simulink model "magnes_bb"  (R2015a)
settings: Solver=ode3  StartTime=0.0  StopTime=0.001  FixedStep=0.00001  RelTol=1e-3
settings Model: Creator=Student  LastModifiedBy=lenovo

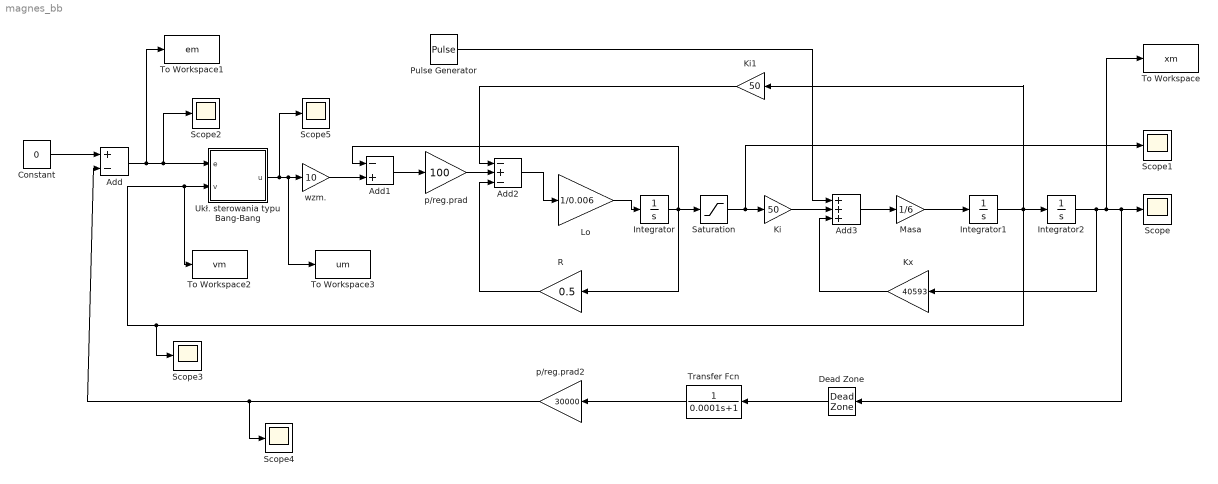
== system magnes_bb ==
  Add : Sum  Inputs=+-
  Add1 : Sum  Inputs=-+
  Add2 : Sum  Inputs=-+-
  Add3 : Sum  Inputs=+++
  Constant : Constant  Value=0
  Dead Zone : DeadZone  LowerValue=-1e-6  UpperValue=1e-6  SaturateOnIntegerOverflow=on
  Integrator : Integrator
  Integrator1 : Integrator
  Integrator2 : Integrator
  Ki : Gain  Gain=50
  Ki1 : Gain  Gain=50
  Kx : Gain  Gain=40593
  Lo : Gain  Gain=1/0.006
  Masa : Gain  Gain=1/6
  Pulse Generator : DiscretePulseGenerator  PulseType=Time based  Amplitude=6*9.81*0.5  Period=0.1  PulseWidth=50  PhaseDelay=0.2
  R : Gain  Gain=0.5
  Saturation : Saturate  UpperLimit=10  LowerLimit=-10
  Scope{,1..5} (6 alike) : Scope
      Scope settings: YMin=-1.5e-06  YMax=1.5e-06
      Scope2 settings: SaveName=ScopeData2
      Scope3 settings: SaveName=ScopeData3
      Scope4 settings: SaveName=ScopeData4
      Scope5 settings: YMin=0.85063  YMax=0.95303  SaveName=ScopeData5
  To Workspace : ToWorkspace  VariableName=xm  SaveFormat=Timeseries  SampleTime=-1
  To Workspace1 : ToWorkspace  VariableName=em  SaveFormat=Timeseries  SampleTime=-1
  To Workspace2 : ToWorkspace  VariableName=vm  SaveFormat=Timeseries  SampleTime=-1
  To Workspace3 : ToWorkspace  VariableName=um  SaveFormat=Timeseries  SampleTime=-1
  Transfer Fcn : TransferFcn  Denominator=[0.0001 1]
  Ukł. sterowania typu Bang-Bang : Stateflow chart  TreatAsAtomicUnit=on
  p/reg.prad : Gain  Gain=100
  p/reg.prad2 : Gain  Gain=30000
  wzm. : Gain  Gain=10
  wires:
  wzm./1 -> Add1/2
  Add1/1 -> p/reg.prad/1
  Add2/1 -> Lo/1
  p/reg.prad/1 -> Add2/2
  Lo/1 -> Integrator/1
  Integrator/1 -> R/1, Add1/1, Saturation/1
  R/1 -> Add2/3
  Constant/1 -> Add/1
  Add/1 -> To Workspace1/1, Scope2/1, Ukł. sterowania typu Bang-Bang/1(e)
  Saturation/1 -> Scope1/1, Ki/1
  Ki/1 -> Add3/2
  Add3/1 -> Masa/1
  Masa/1 -> Integrator1/1
  Kx/1 -> Add3/3
  Dead Zone/1 -> Transfer Fcn/1
  Transfer Fcn/1 -> p/reg.prad2/1
  p/reg.prad2/1 -> Scope4/1, Add/2
  Integrator2/1 -> Kx/1, To Workspace/1, Dead Zone/1, Scope/1
  Integrator1/1 -> Scope3/1, To Workspace2/1, Ukł. sterowania typu Bang-Bang/2(v), Ki1/1, Integrator2/1
  Pulse Generator/1 -> Add3/1
  Ki1/1 -> Add2/1
  Ukł. sterowania typu Bang-Bang/1(u) -> Scope5/1, To Workspace3/1, wzm./1

== stateflow chart magnes_bb/Ukł. sterowania typu Bang-Bang ==
  state 1
    entry: u=-0.9
  state 2
    entry: u=0.9
  (default) -> 1
  1 -> 2 [order 1] : [e>=0]
  1 -> 2 [order 2] : [v<=-0.001]
  2 -> 1 [order 2] : [e<=0]
  2 -> 1 [order 1] : [v>=0.001]
  data: e input; u output; v input
